simulink model "System"  (R2016b)
settings: Solver=VariableStepAuto  StartTime=0.0  StopTime=10  RelTol=1e-3
values from neighbouring files (symbols this model uses):
  g = 10    [Simulink.m]
  Ib = (2/5)*mb*rb^2    (= 1.6)    [Simulink.m]
  mb = 1    [Simulink.m]
  rb = 2    [Simulink.m]
settings Model: Creator=Ashraf  LastModifiedBy=Ashraf

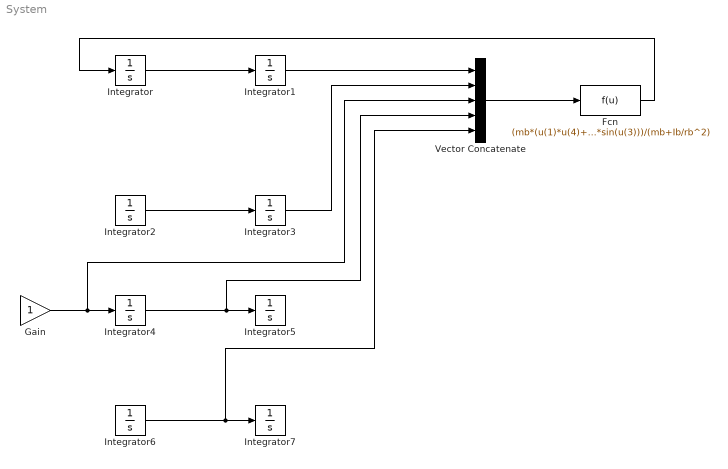
== system System ==
  Fcn : Fcn  Expr=(mb*(u(1)*u(4)+u(2)*u(5))*u(3)-mb*g*sin(u(3)))/(mb+Ib/rb^2)
  Gain : Gain
  Integrator{,1..7} (8 alike) : Integrator
  Vector Concatenate : Concatenate  NumInputs=5
  wires:
  Integrator1/1 -> Vector Concatenate/1
  Integrator3/1 -> Vector Concatenate/2
  Vector Concatenate/1 -> Fcn/1
  Fcn/1 -> Integrator/1
  Gain/1 -> Vector Concatenate/3, Integrator4/1
  Integrator4/1 -> Vector Concatenate/4, Integrator5/1
  Integrator6/1 -> Integrator7/1, Vector Concatenate/5
  Integrator/1 -> Integrator1/1
  Integrator2/1 -> Integrator3/1
